simulink model "model"  (R2013a)
settings: Solver=ode45  StartTime=0.0  StopTime=10.0  RelTol=1e-3
values from neighbouring files (symbols this model uses):
  cp = 1000    [skrypt.m]
  Cv1 = cp*gp*V1    (= 90000)    [skrypt.m]
  Cv2 = cp*gp*V2    (= 144000)    [skrypt.m]
  czas_skoku = 300    [skrypt.m]
  dfk = 0    [skrypt.m]
  dTkz = 0    [skrypt.m]
  dTzew = 0    [skrypt.m]
  fk = fkN*0.5    (= 0.194444444444)    [skrypt.m]
  gp = 1.2    [skrypt.m]
  K0 = (cp*gp*fkN*0.7*(TkzN - T1N)) / (T1N - T2N)    (= 653.333333333)    [skrypt.m]
  K1 = (cp*gp*fkN*0.3*(TkzN-T1N)) / (T1N - TzewN)    (= 35)    [skrypt.m]
  K2 = ((cp*gp*fkN + K0)*(T1N-T2N)) / (T2N - TzewN)    (= 160)    [skrypt.m]
  T10 = (cp*gp*fk*Tkz + K1*Tzew + ((K0*K2*Tzew)/(K0+K2+cp*gp*fk))) / (cp*gp*fk + K1 + K0 - ((K0*(K0+cp*gp*fk))/(K0+K2+cp*gp*fk)))    [skrypt.m]
  T20 = ((K0+cp*gp*fk)*T10 + K2*Tzew) / (K0 + cp*gp*fk + K2)    [skrypt.m]
  Tkz = TkzN    (= 30)    [skrypt.m]
  Tzew = TzewN+i*5    [skrypt.m]
settings Model: Creator=LAB320-1552  LastModifiedBy=LAB320-1552

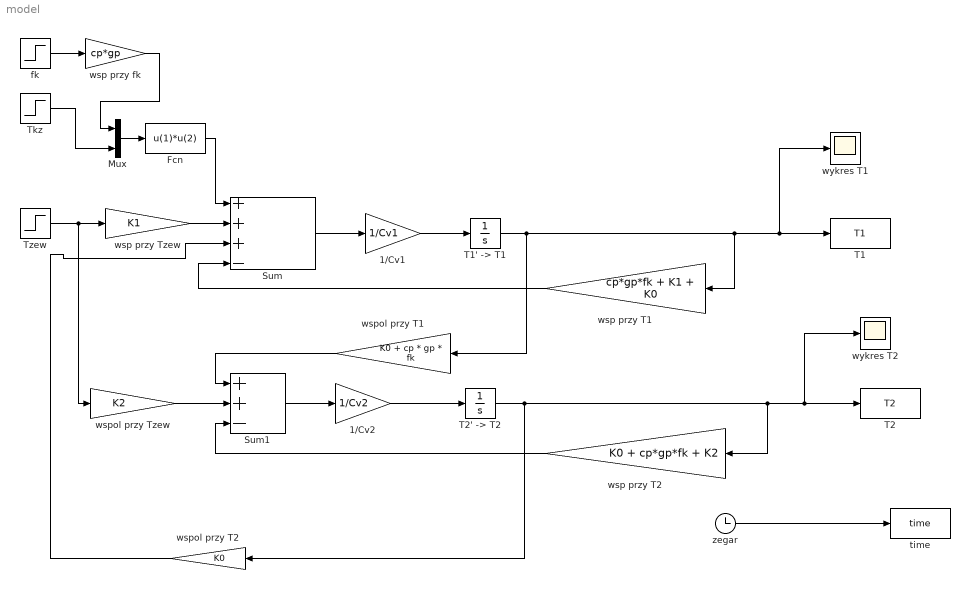
== system model ==
  1/Cv1 : Gain  Gain=1/Cv1
  1/Cv2 : Gain  Gain=1/Cv2
  Fcn : Fcn  Expr=u(1)*u(2)
  Mux : Mux  Inputs=2
  Sum : Sum  Inputs=+|+|+|-
  Sum1 : Sum  Inputs=+|+|-
  T1 : ToWorkspace  VariableName=T1  SampleTime=-1
  "T1' -> T1" : Integrator  InitialCondition=T10
  T2 : ToWorkspace  VariableName=T2  SampleTime=-1
  "T2' -> T2" : Integrator  InitialCondition=T20
  Tkz : Step  Time=czas_skoku  Before=Tkz  After=Tkz+dTkz  SampleTime=0
  Tzew : Step  Time=czas_skoku  Before=Tzew  After=Tzew+dTzew  SampleTime=0
  fk : Step  Time=czas_skoku  Before=fk  After=fk+dfk  SampleTime=0
  time : ToWorkspace  VariableName=time  SampleTime=-1
  wsp przy T1 : Gain  Gain=cp*gp*fk + K1 + K0
  wsp przy T2 : Gain  Gain=K0 + cp*gp*fk + K2
  wsp przy Tzew : Gain  Gain=K1
  wsp przy fk : Gain  Gain=cp*gp
  wspol przy T1 : Gain  Gain=K0 + cp * gp * fk
  wspol przy T2 : Gain  Gain=K0
  wspol przy Tzew : Gain  Gain=K2
  wykres T1 : Scope
  wykres T2 : Scope
  zegar : Clock
  wires:
  1/Cv1/1 -> "T1' -> T1"/1
  Sum/1 -> 1/Cv1/1
  "T1' -> T1"/1 -> wsp przy T1/1, wykres T1/1, T1/1, wspol przy T1/1
  wsp przy Tzew/1 -> Sum/2
  zegar/1 -> time/1
  wspol przy Tzew/1 -> Sum1/2
  wspol przy T1/1 -> Sum1/1
  Sum1/1 -> 1/Cv2/1
  1/Cv2/1 -> "T2' -> T2"/1
  "T2' -> T2"/1 -> wsp przy T2/1, wykres T2/1, T2/1, wspol przy T2/1
  wspol przy T2/1 -> Sum/3
  fk/1 -> wsp przy fk/1
  wsp przy T1/1 -> Sum/4
  wsp przy T2/1 -> Sum1/3
  Tzew/1 -> wspol przy Tzew/1, wsp przy Tzew/1
  wsp przy fk/1 -> Mux/1
  Tkz/1 -> Mux/2
  Mux/1 -> Fcn/1
  Fcn/1 -> Sum/1
